simulink model "forcecontrol"  (R2019a)
settings: Solver=VariableStepAuto  StartTime=0.0  StopTime=5  FixedStep=0.01  RelTol=1e-3
undefined symbols (not defined in the file or in its folder): KI, KP, KV
settings Model: Creator=JanAriel  LastModifiedBy=JanAriel

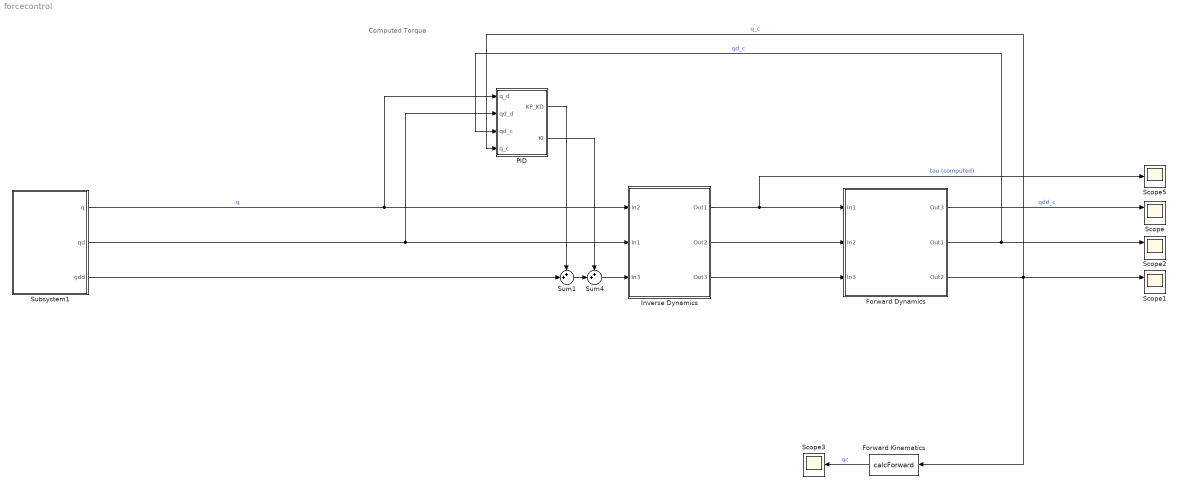
== system forcecontrol ==
  note: Computed Torque
  Forward Dynamics : Subsystem
  Forward Kinematics : MATLABFcn  MATLABFcn=calcForward  Output1D=off
  Inverse Dynamics : Subsystem
  PID : Subsystem
  Scope : Scope  NumInputPorts=2
  Scope1 : Scope  NumInputPorts=2
  Scope2 : Scope  NumInputPorts=2
  Scope3 : Scope
  Scope5 : Scope
  Subsystem1 : Subsystem
  Sum1 : Sum  Inputs=++|
  Sum4 : Sum  Inputs=++|
  wires:
  Inverse Dynamics/1(Out1) -> Forward Dynamics/1(In1), Scope5/1  "tau (computed)"
  Forward Dynamics/1(Out3) -> Scope/1  "qdd_c"
  Forward Dynamics/3(Out2) -> Forward Kinematics/1, PID/4(q_c), Scope1/1  "q_c"
  Subsystem1/2(qd) -> PID/2(qd_d), Inverse Dynamics/2(In1)
  Forward Dynamics/2(Out1) -> PID/3(qd_c), Scope2/1  "qd_c"
  Sum1/1 -> Sum4/2
  Sum4/1 -> Inverse Dynamics/3(In3)
  Subsystem1/1(q) -> PID/1(q_d), Inverse Dynamics/1(In2)  "q"
  Subsystem1/3(qdd) -> Sum1/2
  Inverse Dynamics/2(Out2) -> Forward Dynamics/2(In2)
  Inverse Dynamics/3(Out3) -> Forward Dynamics/3(In3)
  PID/1(KP_KD) -> Sum1/1
  PID/2(KI) -> Sum4/1
  Forward Kinematics/1 -> Scope3/1  "qc"

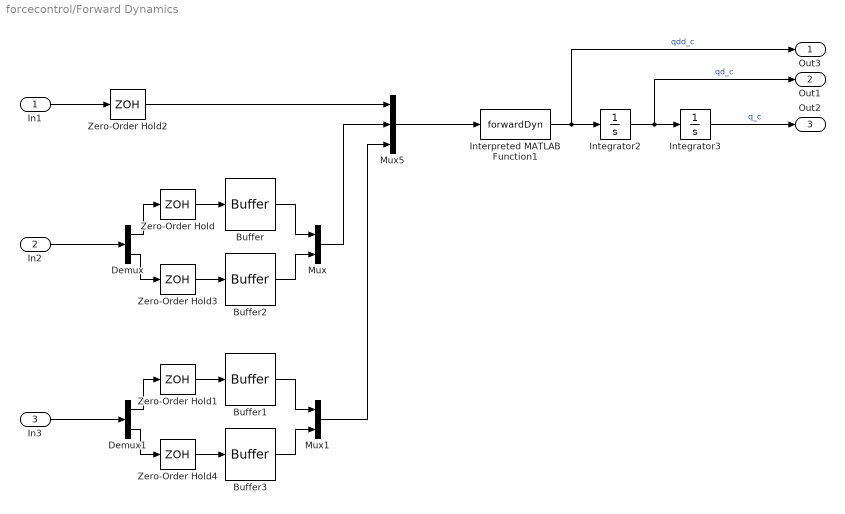
== system forcecontrol/Forward Dynamics ==
  In1 : Inport
  In2 : Inport  Port=2
  In3 : Inport  Port=3
  Buffer{,1..3} (4 alike) : Buffer  N=2  OutputFrames=off
  Demux : Demux  Outputs=2
  Demux1 : Demux  Outputs=2
  Integrator2 : Integrator
  Integrator3 : Integrator
  Interpreted MATLAB Function1 : MATLABFcn  MATLABFcn=forwardDyn  Output1D=off
  Mux : Mux  Inputs=2
  Mux1 : Mux  Inputs=2
  Mux5 : Mux  Inputs=3
  Zero-Order Hold{,1..4} (5 alike) : ZeroOrderHold  SampleTime=0.01
  Out3 : Outport
  Out1 : Outport  Port=2
  Out2 : Outport  Port=3
  wires:
  Integrator2/1 -> Out1/1, Integrator3/1  "qd_c"
  Integrator3/1 -> Out2/1  "q_c"
  Interpreted MATLAB Function1/1 -> Out3/1, Integrator2/1  "qdd_c"
  Mux5/1 -> Interpreted MATLAB Function1/1
  Zero-Order Hold/1 -> Buffer/1
  In1/1 -> Zero-Order Hold2/1
  Zero-Order Hold2/1 -> Mux5/1
  In2/1 -> Demux/1
  Zero-Order Hold3/1 -> Buffer2/1
  Demux/2 -> Zero-Order Hold3/1
  Demux/1 -> Zero-Order Hold/1
  In3/1 -> Demux1/1
  Zero-Order Hold4/1 -> Buffer3/1
  Demux1/1 -> Zero-Order Hold1/1
  Zero-Order Hold1/1 -> Buffer1/1
  Demux1/2 -> Zero-Order Hold4/1
  Buffer/1 -> Mux/1
  Buffer2/1 -> Mux/2
  Buffer3/1 -> Mux1/2
  Buffer1/1 -> Mux1/1
  Mux/1 -> Mux5/2
  Mux1/1 -> Mux5/3

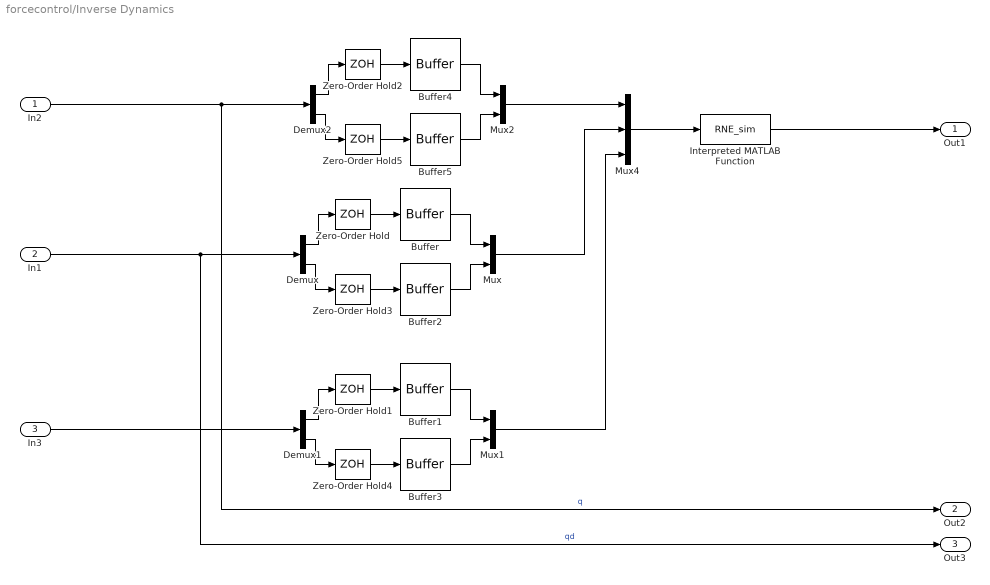
== system forcecontrol/Inverse Dynamics ==
  In2 : Inport
  In1 : Inport  Port=2
  In3 : Inport  Port=3
  Buffer{,1..5} (6 alike) : Buffer  N=2  OutputFrames=off
  Demux : Demux  Outputs=2
  Demux1 : Demux  Outputs=2
  Demux2 : Demux  Outputs=2
  Interpreted MATLAB Function : MATLABFcn  MATLABFcn=RNE_sim  Output1D=off
  Mux : Mux  Inputs=2
  Mux1 : Mux  Inputs=2
  Mux2 : Mux  Inputs=2
  Mux4 : Mux  Inputs=3
  Zero-Order Hold{,1..5} (6 alike) : ZeroOrderHold  SampleTime=0.01
  Out1 : Outport
  Out2 : Outport  Port=2
  Out3 : Outport  Port=3
  wires:
  In1/1 -> Demux/1, Out3/1  "qd"
  Mux4/1 -> Interpreted MATLAB Function/1
  Interpreted MATLAB Function/1 -> Out1/1
  Demux1/1 -> Zero-Order Hold1/1
  Mux1/1 -> Mux4/3
  Buffer/1 -> Mux/1
  Mux/1 -> Mux4/2
  Zero-Order Hold1/1 -> Buffer1/1
  Buffer3/1 -> Mux1/2
  Zero-Order Hold3/1 -> Buffer2/1
  Buffer1/1 -> Mux1/1
  Demux/2 -> Zero-Order Hold3/1
  In3/1 -> Demux1/1
  Buffer2/1 -> Mux/2
  Zero-Order Hold4/1 -> Buffer3/1
  Demux/1 -> Zero-Order Hold/1
  Demux1/2 -> Zero-Order Hold4/1
  Zero-Order Hold/1 -> Buffer/1
  Buffer5/1 -> Mux2/2
  Demux2/1 -> Zero-Order Hold2/1
  Zero-Order Hold5/1 -> Buffer5/1
  Buffer4/1 -> Mux2/1
  Mux2/1 -> Mux4/1
  Demux2/2 -> Zero-Order Hold5/1
  Zero-Order Hold2/1 -> Buffer4/1
  In2/1 -> Out2/1, Demux2/1  "q"

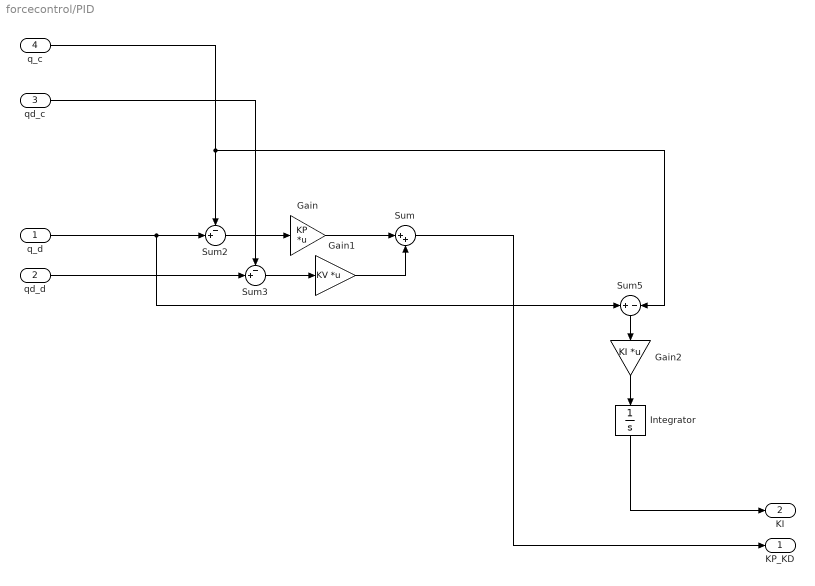
== system forcecontrol/PID ==
  q_d : Inport
  qd_d : Inport  Port=2
  qd_c : Inport  Port=3
  q_c : Inport  Port=4
  Gain : Gain  Gain=KP  Multiplication=Matrix(K*u) (u vector)
  Gain1 : Gain  Gain=KV  Multiplication=Matrix(K*u) (u vector)
  Gain2 : Gain  Gain=KI  Multiplication=Matrix(K*u) (u vector)
  Integrator : Integrator
  Sum : Sum  Inputs=|++
  Sum2 : Sum  Inputs=-+|
  Sum3 : Sum  Inputs=-+|
  Sum5 : Sum  Inputs=+-
  KP_KD : Outport
  KI : Outport  Port=2
  wires:
  q_c/1 -> Sum5/2, Sum2/1
  Sum5/1 -> Gain2/1
  q_d/1 -> Sum2/2, Sum5/1
  Sum2/1 -> Gain/1
  Sum3/1 -> Gain1/1
  Gain2/1 -> Integrator/1
  Gain1/1 -> Sum/2
  Gain/1 -> Sum/1
  qd_c/1 -> Sum3/1
  Sum/1 -> KP_KD/1
  Integrator/1 -> KI/1
  qd_d/1 -> Sum3/2

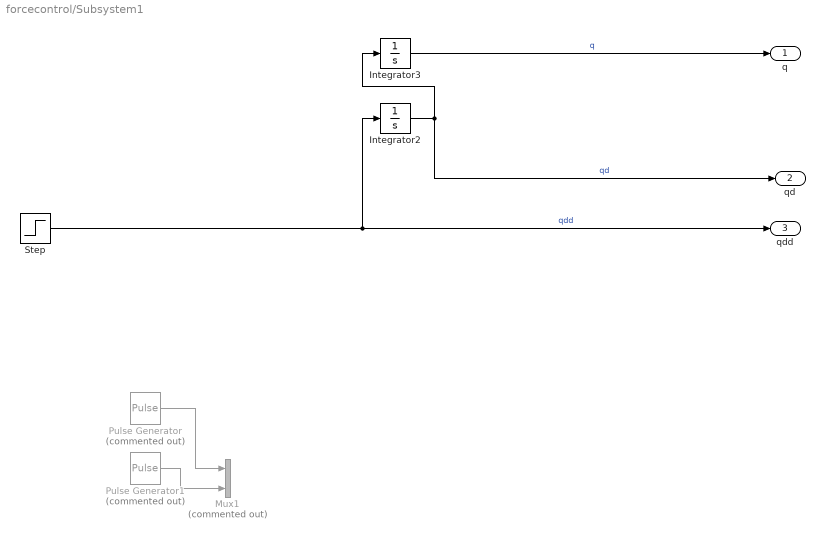
== system forcecontrol/Subsystem1 ==
  Integrator2 : Integrator
  Integrator3 : Integrator
  Mux1 : Mux  Commented=on  Inputs=2
  Pulse Generator : DiscretePulseGenerator  Commented=on  PulseType=Time based  PulseWidth=5
  Pulse Generator1 : DiscretePulseGenerator  Commented=on  PulseType=Time based  PulseWidth=5
  Step : Step  Before=[0;0]  After=[0.35;0.35]  SampleTime=0  VectorParams1D=off
  q : Outport
  qd : Outport  Port=2
  qdd : Outport  Port=3
  wires:
  Integrator2/1 -> qd/1, Integrator3/1  "qd"
  Step/1 -> Integrator2/1, qdd/1  "qdd"
  Integrator3/1 -> q/1  "q"
  Pulse Generator1/1 -> Mux1/2
  Pulse Generator/1 -> Mux1/1
